simulink model "Pend_Simscape_Closedloop"  (R2017a)
settings: Solver=FixedStepAuto  StartTime=0.0  StopTime=15  FixedStep=0.01  RelTol=1e-3
model workspace (MAT data in the model file):
  I = 0.006
  M = 0.5
  b = 0.1
  g = 9.81
  l = 0.3
  m = 0.2
libraries: mblibv1 x13, simulink x2
settings Model: Creator=sansh  LastModifiedBy=proko
settings SimMechanicsCC: VisDuringSimulation=on

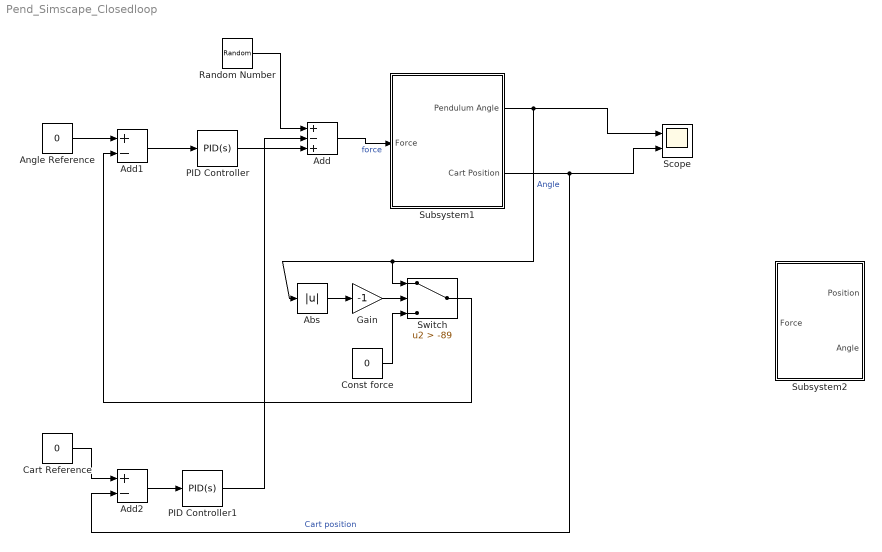
== system Pend_Simscape_Closedloop ==
  Abs : Abs
  Add : Sum  Inputs=+-+
  Add1 : Sum  Inputs=+-
  Add2 : Sum  Inputs=+-
  Angle Reference : Constant  Value=0
  Cart Reference : Constant  Value=0
  Const force : Constant  Value=0
  Gain : Gain  Gain=-1
  PID Controller : simulink/Continuous/PID Controller  Controller=PID  TimeDomain=Continuous-time  SampleTime=-1  IntegratorMethod=Forward Euler  FilterMethod=Forward Euler  Form=Parallel  UseFilter=on  ControllerParametersSource=internal  P=1  I=1  D=0.1  N=100  InitialConditionSource=internal  InitialConditionForIntegrator=0  InitialConditionForFilter=0  ExternalReset=none  LimitOutput=off  UpperSaturationLimit=inf  LowerSaturationLimit=-inf  LinearizeAsGain=on  AntiWindupMode=none  Kb=1  TrackingMode=off  Kt=1  PParamMin=[]  PParamMax=[]  IParamMin=[]  IParamMax=[]  DParamMin=[]  DParamMax=[]  NParamMin=[]  NParamMax=[]  KbParamMin=[]  KbParamMax=[]  KtParamMin=[]  KtParamMax=[]  POutMin=[]  POutMax=[]  IOutMin=[]  IOutMax=[]  DOutMin=[]  DOutMax=[]  NOutMin=[]  NOutMax=[]  KbOutMin=[]  KbOutMax=[]  KtOutMin=[]  KtOutMax=[]  IntegratorOutMin=[]  IntegratorOutMax=[]  FilterOutMin=[]  FilterOutMax=[]  SumOutMin=[]  SumOutMax=[]  SumI1OutMin=[]  SumI1OutMax=[]  SumI2OutMin=[]  SumI2OutMax=[]  SumI3OutMin=[]  SumI3OutMax=[]  SumDOutMin=[]  SumDOutMax=[]  SaturationOutMin=[]  SaturationOutMax=[]  IntegratorContinuousStateAttributes=''  IntegratorStateMustResolveToSignalObject=off  IntegratorRTWStateStorageClass=Auto  FilterContinuousStateAttributes=''  FilterStateMustResolveToSignalObject=off  FilterRTWStateStorageClass=Auto  DifferentiatorICPrevScaledInput=0  DifferentiatorOutMin=[]  DifferentiatorOutMax=[]  InitialConditionSetting=State (most efficient)
  PID Controller1 : simulink/Continuous/PID Controller  Controller=PID  TimeDomain=Continuous-time  SampleTime=-1  IntegratorMethod=Forward Euler  FilterMethod=Forward Euler  Form=Parallel  UseFilter=on  ControllerParametersSource=internal  P=10  I=3  D=3  N=100  InitialConditionSource=internal  InitialConditionForIntegrator=0  InitialConditionForFilter=0  ExternalReset=none  LimitOutput=off  UpperSaturationLimit=inf  LowerSaturationLimit=-inf  LinearizeAsGain=on  AntiWindupMode=none  Kb=1  TrackingMode=off  Kt=1  PParamMin=[]  PParamMax=[]  IParamMin=[]  IParamMax=[]  DParamMin=[]  DParamMax=[]  NParamMin=[]  NParamMax=[]  KbParamMin=[]  KbParamMax=[]  KtParamMin=[]  KtParamMax=[]  POutMin=[]  POutMax=[]  IOutMin=[]  IOutMax=[]  DOutMin=[]  DOutMax=[]  NOutMin=[]  NOutMax=[]  KbOutMin=[]  KbOutMax=[]  KtOutMin=[]  KtOutMax=[]  IntegratorOutMin=[]  IntegratorOutMax=[]  FilterOutMin=[]  FilterOutMax=[]  SumOutMin=[]  SumOutMax=[]  SumI1OutMin=[]  SumI1OutMax=[]  SumI2OutMin=[]  SumI2OutMax=[]  SumI3OutMin=[]  SumI3OutMax=[]  SumDOutMin=[]  SumDOutMax=[]  SaturationOutMin=[]  SaturationOutMax=[]  IntegratorContinuousStateAttributes=''  IntegratorStateMustResolveToSignalObject=off  IntegratorRTWStateStorageClass=Auto  FilterContinuousStateAttributes=''  FilterStateMustResolveToSignalObject=off  FilterRTWStateStorageClass=Auto  DifferentiatorICPrevScaledInput=0  DifferentiatorOutMin=[]  DifferentiatorOutMax=[]  InitialConditionSetting=State (most efficient)
  Random Number : RandomNumber  Mean=10  Variance=100  SampleTime=1
  Scope : Scope  NumInputPorts=2
  Subsystem1 : Subsystem
  Subsystem2 : Subsystem
  Switch : Switch  Criteria=u2 > Threshold  Threshold=-89
  wires:
  Subsystem1/1(Pendulum Angle) -> Abs/1, Switch/1, Scope/1  "Angle"
  Add1/1 -> PID Controller/1
  PID Controller/1 -> Add/3
  Angle Reference/1 -> Add1/1
  Add/1 -> Subsystem1/1(Force)  "force"
  Subsystem1/2(Cart Position) -> Add2/2, Scope/2  "Cart position"
  Switch/1 -> Add1/2
  Abs/1 -> Gain/1
  Gain/1 -> Switch/2
  Const force/1 -> Switch/3
  PID Controller1/1 -> Add/2
  Cart Reference/1 -> Add2/1
  Add2/1 -> PID Controller1/1
  Random Number/1 -> Add/1

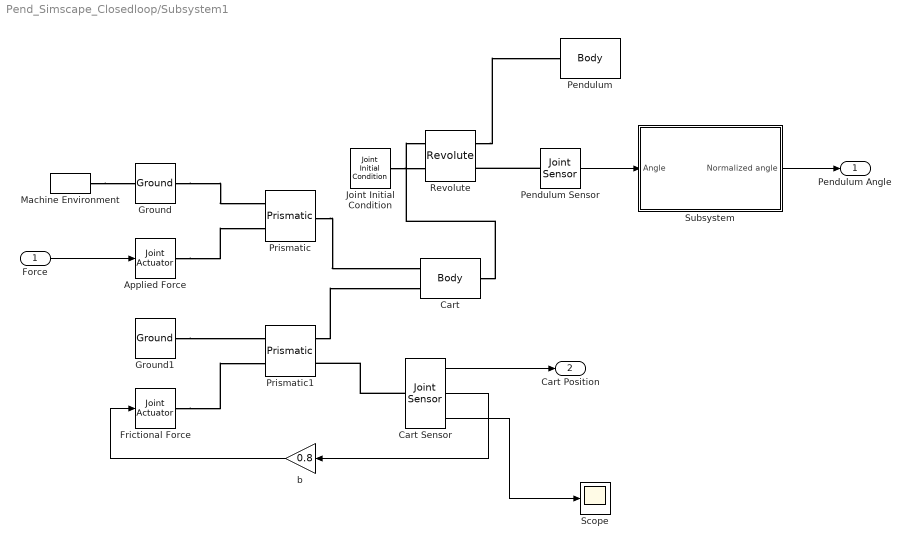
== system Pend_Simscape_Closedloop/Subsystem1 ==
  Force : Inport
  " Pendulum Sensor" : mblibv1/Sensors &  Actuators/Joint Sensor  UpdateFromCAD=off  PhysicalDomain=Mechanical  PortType=blob  Muxed=on  Pose=off  Angle=on  AngleUnits=deg  ArcVelocity=off  ArcVelocityUnits=deg/s  ArcAcceleration=off  ArcAccelerationUnits=deg/s^2  CoordPosition=on  CoordPositionUnits=m  Velocity=off  VelocityUnits=m/s  Acceleration=off  AccelerationUnits=m/s^2  Quaternion=on  QuaternionDT=off  QuaternionDDT=off  QuaternionUnits=off  OutputVector=[1]  ActiveIO=on  Width=1  DialogClass=MechanicalSensorBlock  Primitive=R1  Force=off  ForceUnits=N  Torque=off  TorqueUnits=N*m  ReferenceFrame=Absolute (World)  ReactionSensedSide=Base  ReactionReferenceFrame=Absolute (World)  ReactionForce=off  ReactionForceUnits=N  ReactionMoment=off  ReactionMomentUnits=N*m
      settings: SourceProductName=Simscape Multibody  SourceProductBaseCode=MS
  Applied Force : mblibv1/Sensors &  Actuators/Joint Actuator  UpdateFromCAD=off  PhysicalDomain=Mechanical  PortType=blob  ActuationStyle=Force  AngleUnits=deg  ArcVelocityUnits=deg/s  ArcAccelerationUnits=deg/s^2  CoordPositionUnits=m  VelocityUnits=m/s  AccelerationUnits=m/s^2  ForceUnits=N  TorqueUnits=N-m  ActiveIO=on  Width=1  DialogClass=MechanicalActuatorBlock  Primitive=P1  ReferenceFrame=Absolute (World)
      settings: SourceProductName=Simscape Multibody  SourceProductBaseCode=MS
  Cart : mblibv1/Bodies/Body  LConnTagsString=CS1|CS2  RConnTagsString=CS3  UpdateFromCAD=off  DialogClass=MechanicalBodyBlock  Mass=0.5  MassUnits=kg  InertiaUnits=kg*m^2  Inertia=eye(3)  Shape=Cylinder  ShapeDims=[1 1]  ShapeUnits=m  ShapeUse=false  Density=1  DensityUnits=kg/m^3  DensityUse=false  GraphicsMode=MACHINE_DEFAULT  BodyColorSelMode=MACHINE_DEFAULT  BodyColor=[1 0 0]  AttachedToCS=CG  CG=Left$CG$[0 0 0]$WORLD$WORLD$m$[0 0 0]$Euler X-Y-Z$deg$WORLD$false$none  WorkingFrames=Left$CS1$[-1 0 0]$CG$CG$m$[0 0 0]$Euler X-Y-Z$deg$WORLD$true$none#Left$CS2$[0 0 0]$CG$CG$m$[0 0 0]$Euler X-Y-Z$deg$WORLD$true$none#Right$CS3$[0 0.5 0]$CG$CG$m$[0 0 0]$Euler X-Y-Z$deg$WORLD$true$none#Right$CS4$[-1 0.5 0]$CG$CG$m$[0 0 0]$Euler X-Y-Z$deg$WORLD$false$none#Right$CS5$[-1 -0.5 0]$CG$CG$m$[0 0 0]$Euler X-Y-Z$deg$WORLD$false$none#Right$CS6$[1 -0.5 0]$CG$CG$m$[0 0 0]$Euler X-Y-Z$deg$WORLD$false$none#Right$CS7$[1 0.5 0]$CG$CG$m$[0 0 0]$Euler X-Y-Z$deg$WORLD$false$none  CGPos=[0 0 0]  CGRot=[0 0 0]  CS0Pos=[]  CS0Rot=[]  CS1Pos=[-1 0 0]  CS1Rot=[0 0 0]  CS2Pos=[0 0 0]  CS2Rot=[0 0 0]  CS3Pos=[0 0.5 0]  CS3Rot=[0 0 0]  CS4Pos=[-1 0.5 0]  CS4Rot=[0 0 0]  CS5Pos=[-1 -0.5 0]  CS5Rot=[0 0 0]  CS6Pos=[1 -0.5 0]  CS6Rot=[0 0 0]  CS7Pos=[1 0.5 0]  CS7Rot=[0 0 0]  CS8Pos=[]  CS8Rot=[]  CS9Pos=[]  CS9Rot=[]  CS10Pos=[]  CS10Rot=[]  CS11Pos=[]  CS11Rot=[]  CS12Pos=[]  CS12Rot=[]  CS13Pos=[]  CS13Rot=[]  CS14Pos=[]  CS14Rot=[]  CS15Pos=[]  CS15Rot=[]  CS16Pos=[]  CS16Rot=[]  CS17Pos=[]  CS17Rot=[]  CS18Pos=[]  CS18Rot=[]  CS19Pos=[]  CS19Rot=[]  CS20Pos=[]  CS20Rot=[]
      settings: SourceProductName=Simscape Multibody  SourceProductBaseCode=MS
  Cart Sensor : mblibv1/Sensors &  Actuators/Joint Sensor  UpdateFromCAD=off  PhysicalDomain=Mechanical  PortType=blob  Muxed=off  Pose=off  Angle=on  AngleUnits=deg  ArcVelocity=off  ArcVelocityUnits=deg/s  ArcAcceleration=off  ArcAccelerationUnits=deg/s^2  CoordPosition=on  CoordPositionUnits=m  Velocity=on  VelocityUnits=m/s  Acceleration=on  AccelerationUnits=m/s^2  Quaternion=on  QuaternionDT=off  QuaternionDDT=off  QuaternionUnits=off  OutputVector=[1]  ActiveIO=on  Width=3  DialogClass=MechanicalSensorBlock  Primitive=P1  Force=off  ForceUnits=N  Torque=off  TorqueUnits=N*m  ReferenceFrame=Absolute (World)  ReactionSensedSide=Base  ReactionReferenceFrame=Absolute (World)  ReactionForce=off  ReactionForceUnits=N  ReactionMoment=off  ReactionMomentUnits=N*m
      settings: SourceProductName=Simscape Multibody  SourceProductBaseCode=MS
  Frictional Force : mblibv1/Sensors &  Actuators/Joint Actuator  UpdateFromCAD=off  PhysicalDomain=Mechanical  PortType=blob  ActuationStyle=Force  AngleUnits=deg  ArcVelocityUnits=deg/s  ArcAccelerationUnits=deg/s^2  CoordPositionUnits=m  VelocityUnits=m/s  AccelerationUnits=m/s^2  ForceUnits=N  TorqueUnits=N-m  ActiveIO=on  Width=1  DialogClass=MechanicalActuatorBlock  Primitive=P1  ReferenceFrame=Absolute (World)
      settings: SourceProductName=Simscape Multibody  SourceProductBaseCode=MS
  Ground : mblibv1/Bodies/Ground  UpdateFromCAD=off  LeftPortType=env  RightPortType=workingframe  PhysicalDomain=Mechanical  DialogClass=GroundBlock  CoordPosition=[0 0 0]  CoordPositionUnits=m  StateVectorMgrId=0  MachineId=[1 0]  ShowEnvPort=on  ParameterChecksum=[71100045, 305287200, 426167544, 2566686685]  TopologyChecksum=[1397313767, 1010147589, 575654971, 604440580]
      settings: SourceProductName=Simscape Multibody  SourceProductBaseCode=MS
  Ground1 : mblibv1/Bodies/Ground  UpdateFromCAD=off  LeftPortType=env  RightPortType=workingframe  PhysicalDomain=Mechanical  DialogClass=GroundBlock  CoordPosition=[0 0 0]  CoordPositionUnits=m  StateVectorMgrId=-1  MachineId=[0 0]  ShowEnvPort=off  ParameterChecksum=[0 0 0 0]  TopologyChecksum=[0 0 0 0]
      settings: SourceProductName=Simscape Multibody  SourceProductBaseCode=MS
  Joint Initial Condition : mblibv1/Sensors &  Actuators/Joint Initial Condition  UpdateFromCAD=off  LeftPortType=blob  RightPortType=blob  PhysicalDomain=mechanical  DialogClass=InitialConditionBlock  InitialConditions=P1$false$0$m$deg$0$m/s$deg/s#P2$false$0$m$deg$0$m/s$deg/s#P3$false$0$m$deg$0$m/s$deg/s#R1$true$45$m$deg$0$m/s$deg/s#R2$false$0$m$deg$0$m/s$deg/s#R3$false$0$m$deg$0$m/s$deg/s#S$false$0$m$deg$0$m/s$deg/s  P1PIC=0  P1VIC=0  P2PIC=0  P2VIC=0  P3PIC=0  P3VIC=0  R1PIC=45  R1VIC=0  R2PIC=0  R2VIC=0  R3PIC=0  R3VIC=0  SPIC=0  SVIC=0
      settings: SourceProductName=Simscape Multibody  SourceProductBaseCode=MS
  Machine Environment : mblibv1/Bodies/Machine Environment  PortType=env  PhysicalDomain=Mechanical  DialogTemplateClass=MECH.MachineEnvironment  SyncWhenCopied=off  Gravity=[0 -9.81 0]  GravityUnits=m/s^2  GravityAsSignal=off  Dimensionality=Auto-detect  AnalysisType=Forward dynamics  LinearAssemblyTolerance=1e-3  LinearAssemblyToleranceUnits=m  AngularAssemblyTolerance=1e-3  AngularAssemblyToleranceUnits=rad  ConstraintSolverType=Stabilizing  ConstraintRelTolerance=1e-4  ConstraintAbsTolerance=1e-4  UseRobustSingularityHandling=off  RedundancyAnalysisToleranceType=Automatically select tolerance  RedundancyAnalysisTolerance=1e-14  StatePerturbationType=Fixed  PerturbationSize=1e-5  VisualizeMachine=on  BodyVisualizationType=Use model default body geometries  BodyColorSelMode=Use model default  DefaultBodyColor=[1 0 0]
      settings: SourceProductName=Simscape Multibody  SourceProductBaseCode=MS
  Pendulum : mblibv1/Bodies/Body  LConnTagsString=CS1  UpdateFromCAD=off  DialogClass=MechanicalBodyBlock  Mass=0.2  MassUnits=kg  InertiaUnits=kg*m^2  Inertia=0.006*eye(3)  Shape=Cylinder  ShapeDims=[1 1]  ShapeUnits=m  ShapeUse=false  Density=1  DensityUnits=kg/m^3  DensityUse=false  GraphicsMode=MACHINE_DEFAULT  BodyColorSelMode=MACHINE_DEFAULT  BodyColor=[1 0 0]  AttachedToCS=CG  CG=Left$CG$[0 0.3 0]$CS1$CS1$m$[0 0 0]$Euler X-Y-Z$deg$WORLD$false$none  WorkingFrames=Left$CS1$[0 0 0]$Adjoining$Adjoining$m$[0 0 0]$Euler X-Y-Z$deg$WORLD$true$none#Right$CS2$[0.1 0 0]$CS1$CS1$m$[0 0 0]$Euler X-Y-Z$deg$WORLD$false$none#Right$CS3$[-0.1 0 0]$CS1$CS1$m$[0 0 0]$Euler X-Y-Z$deg$WORLD$false$none#Right$CS4$[-0.1 0.6 0]$CS1$CS1$m$[0 0 0]$Euler X-Y-Z$deg$WORLD$false$none#Right$CS5$[0.1 0.6 0]$CS1$CS1$m$[0 0 0]$Euler X-Y-Z$deg$WORLD$false$none  CGPos=[0 0.3 0]  CGRot=[0 0 0]  CS0Pos=[]  CS0Rot=[]  CS1Pos=[0 0 0]  CS1Rot=[0 0 0]  CS2Pos=[0.1 0 0]  CS2Rot=[0 0 0]  CS3Pos=[-0.1 0 0]  CS3Rot=[0 0 0]  CS4Pos=[-0.1 0.6 0]  CS4Rot=[0 0 0]  CS5Pos=[0.1 0.6 0]  CS5Rot=[0 0 0]  CS6Pos=[]  CS6Rot=[]  CS7Pos=[]  CS7Rot=[]  CS8Pos=[]  CS8Rot=[]  CS9Pos=[]  CS9Rot=[]  CS10Pos=[]  CS10Rot=[]  CS11Pos=[]  CS11Rot=[]  CS12Pos=[]  CS12Rot=[]  CS13Pos=[]  CS13Rot=[]  CS14Pos=[]  CS14Rot=[]  CS15Pos=[]  CS15Rot=[]  CS16Pos=[]  CS16Rot=[]  CS17Pos=[]  CS17Rot=[]  CS18Pos=[]  CS18Rot=[]  CS19Pos=[]  CS19Rot=[]  CS20Pos=[]  CS20Rot=[]
      settings: SourceProductName=Simscape Multibody  SourceProductBaseCode=MS
  Prismatic : mblibv1/Joints/Prismatic  LConnTagsString=__newl0|SA1  RConnTagsString=__newr0  UpdateFromCAD=off  NumSAPorts=1  CutJoint=off  MarkAsCut=off  Primitives=prismatic  PrimitiveProps=P1$World$[1 0 0]$prismatic  DialogClass=JointBlock  P1Axis=[1 0 0]
      settings: SourceProductName=Simscape Multibody  SourceProductBaseCode=MS
  Prismatic1 : mblibv1/Joints/Prismatic  LConnTagsString=__newl0|SA1  RConnTagsString=__newr0|SA1  UpdateFromCAD=off  NumSAPorts=2  CutJoint=off  MarkAsCut=off  Primitives=prismatic  PrimitiveProps=P1$World$[1 0 0]$prismatic  DialogClass=JointBlock  P1Axis=[1 0 0]
      settings: SourceProductName=Simscape Multibody  SourceProductBaseCode=MS
  Revolute : mblibv1/Joints/Revolute  LConnTagsString=__newl0|SA1  RConnTagsString=__newr0|SA1  UpdateFromCAD=off  NumSAPorts=2  CutJoint=off  MarkAsCut=off  Primitives=prismatic  PrimitiveProps=R1$World$[0 0 1]$revolute  DialogClass=JointBlock  R1Axis=[0 0 1]
      settings: SourceProductName=Simscape Multibody  SourceProductBaseCode=MS
  Scope : Scope
  Subsystem : Subsystem
  b : Gain  Gain=0.8
  Pendulum Angle : Outport
  Cart Position : Outport  Port=2
  wires:
  Force/1 -> Applied Force/1
  Cart Sensor/2 -> b/1
  b/1 -> Frictional Force/1
  Cart Sensor/1 -> Cart Position/1
  Subsystem/1(Normalized angle) -> Pendulum Angle/1
  " Pendulum Sensor"/1 -> Subsystem/1(Angle)
  Cart Sensor/3 -> Scope/1
  connections:
  Revolute/RConn1 -- Pendulum/LConn1
  Joint Initial Condition/RConn1 -- Revolute/LConn2
  Cart/RConn1 -- Revolute/LConn1
  Machine Environment/RConn1 -- Ground/LConn1
  Prismatic1/RConn1 -- Cart/LConn2
  Ground1/RConn1 -- Prismatic1/LConn1
  Prismatic/RConn1 -- Cart/LConn1
  " Pendulum Sensor"/LConn1 -- Revolute/RConn2
  Cart Sensor/LConn1 -- Prismatic1/RConn2
  Applied Force/RConn1 -- Prismatic/LConn2
  Frictional Force/RConn1 -- Prismatic1/LConn2
  Ground/RConn1 -- Prismatic/LConn1

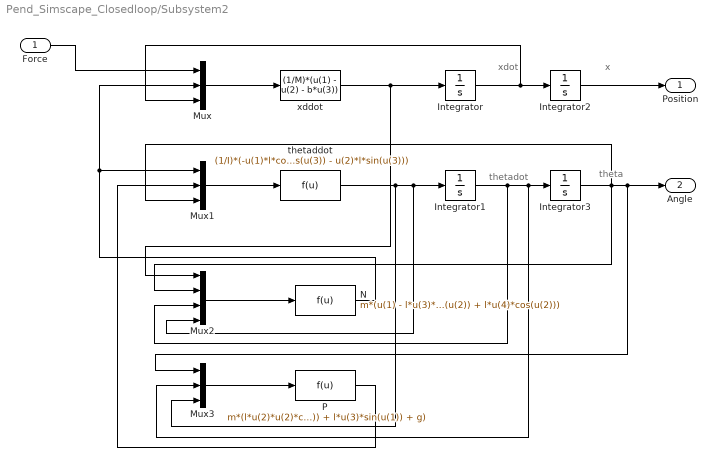
== system Pend_Simscape_Closedloop/Subsystem2 ==
  note: xdot
  note: thetadot
  note: x
  note: theta
  Force : Inport
  Integrator : Integrator  ContinuousStateAttributes='xdot'
  Integrator1 : Integrator  ContinuousStateAttributes='thetadot'
  Integrator2 : Integrator  ContinuousStateAttributes='x'
  Integrator3 : Integrator  InitialCondition=pi  ContinuousStateAttributes='theta'
  Mux : Mux  Inputs=3
  Mux1 : Mux  Inputs=3
  Mux2 : Mux
  Mux3 : Mux  Inputs=3
  N : Fcn  Expr=m*(u(1) - l*u(3)*u(3)*sin(u(2)) + l*u(4)*cos(u(2)))
  P : Fcn  Expr=m*(l*u(2)*u(2)*cos(u(1)) + l*u(3)*sin(u(1)) + g)
  thetaddot : Fcn  Expr=(1/I)*(-u(1)*l*cos(u(3)) - u(2)*l*sin(u(3)))
  xddot : Fcn  Expr=(1/M)*(u(1) - u(2) - b*u(3))
  Position : Outport
  Angle : Outport  Port=2
  wires:
  Integrator3/1 -> Mux3/1, Angle/1, Mux1/3, Mux2/2
  Integrator1/1 -> Integrator3/1, Mux3/2, Mux2/3
  Integrator/1 -> Integrator2/1, Mux/3
  thetaddot/1 -> Integrator1/1, Mux2/4, Mux3/3
  Integrator2/1 -> Position/1
  xddot/1 -> Integrator/1, Mux2/1
  Mux1/1 -> thetaddot/1
  N/1 -> Mux/2, Mux1/1
  Mux3/1 -> P/1
  P/1 -> Mux1/2
  Mux/1 -> xddot/1
  Mux2/1 -> N/1
  Force/1 -> Mux/1

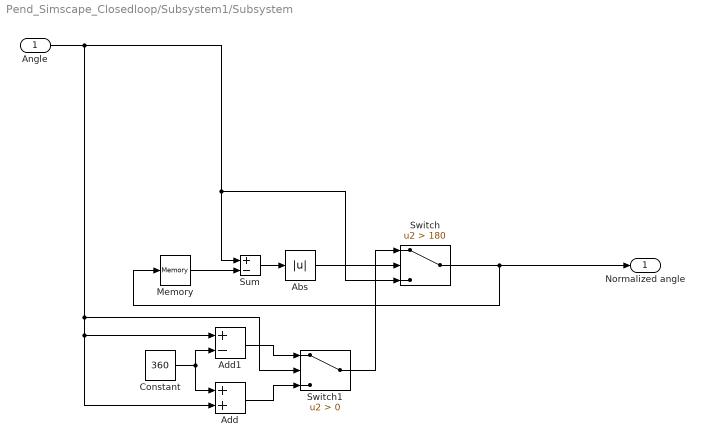
== system Pend_Simscape_Closedloop/Subsystem1/Subsystem ==
  Angle : Inport
  Abs : Abs
  Add : Sum
  Add1 : Sum  Inputs=+-
  Constant : Constant  Value=360
  Memory : Memory  X0=45
  Sum : Sum  Inputs=+-
  Switch : Switch  Criteria=u2 > Threshold  Threshold=180
  Switch1 : Switch  Criteria=u2 > Threshold
  Normalized angle : Outport
  wires:
  Memory/1 -> Sum/2
  Sum/1 -> Abs/1
  Abs/1 -> Switch/2
  Switch/1 -> Memory/1, Normalized angle/1
  Add/1 -> Switch1/3
  Constant/1 -> Add/1, Add1/2
  Add1/1 -> Switch1/1
  Switch1/1 -> Switch/1
  Angle/1 -> Switch1/2, Add/2, Add1/1, Switch/3, Sum/1
